simulink model "VCU_CS75_12_27_test"  (R2014a)
settings: Solver=FixedStepDiscrete  StartTime=0.0  StopTime=25  FixedStep=0.0005  RelTol=1e-3
undefined symbols (not defined in the file): D1, D2, D3, ecucoder_acal, ErrorSumMax1, ErrorSumMax2, ErrorSumMax3, I1, I2, I3, I_SW01_L, LaterlAngleCommand, LDW, P1, P2, P3, RemoteAcclPosition
libraries: simulink x913, ec5744lib x39
(part 22 of 30)

== system VCU_CS75_12_27_test/长安CS75底盘程序，20ms一次/Output/Subsystem/TransmitMessages3/ACC_3D5/ACC_RightTargetType ==
  ACC_RightTargetType : Inport
  ACC_RightTargetTypeRon : Rounding  Operator=round
  ACC_RightTargetType_1sat : Saturate  UpperLimit=224  LowerLimit=0
  ACC_RightTargetType_Convert : DataTypeConversion  OutDataTypeStr=uint8
  ACC_RightTargetType_Convert1 : DataTypeConversion  OutDataTypeStr=uint32
  ACC_RightTargetType_D : Product  Inputs=*/
  ACC_RightTargetType_F : Constant  OutDataTypeStr=single
  ACC_RightTargetType_L : simulink/Logic and Bit Operations/Bitwise Operator  logicop=AND  UseBitMask=on  BitMask=224  BitMaskRealWorld=Stored Integer
  ACC_RightTargetType_O : Constant  Value=0  OutDataTypeStr=single
  ACC_RightTargetType_S : ArithShift  BitShiftNumber=-5
  ACC_RightTargetType_sat : Saturate  UpperLimit=0  LowerLimit=0
  ACC_RightTargetType_st : Sum  Inputs=+-
  Constant{1..2,4..8} (7 alike) : Constant  Value=0  OutDataTypeStr=uint8
  output1 : Outport
  output2 : Outport  Port=2
  output3 : Outport  Port=3
  output4 : Outport  Port=4
  output5 : Outport  Port=5
  output6 : Outport  Port=6
  output7 : Outport  Port=7
  output8 : Outport  Port=8
  wires:
  ACC_RightTargetType/1 -> ACC_RightTargetType_sat/1
  ACC_RightTargetType_sat/1 -> ACC_RightTargetType_st/1
  ACC_RightTargetType_O/1 -> ACC_RightTargetType_st/2
  ACC_RightTargetType_st/1 -> ACC_RightTargetType_D/1
  ACC_RightTargetType_F/1 -> ACC_RightTargetType_D/2
  ACC_RightTargetType_D/1 -> ACC_RightTargetTypeRon/1
  ACC_RightTargetTypeRon/1 -> ACC_RightTargetType_S/1
  ACC_RightTargetType_S/1 -> ACC_RightTargetType_1sat/1
  ACC_RightTargetType_1sat/1 -> ACC_RightTargetType_Convert1/1
  ACC_RightTargetType_Convert1/1 -> ACC_RightTargetType_L/1
  ACC_RightTargetType_L/1 -> ACC_RightTargetType_Convert/1
  ACC_RightTargetType_Convert/1 -> output3/1
  Constant1/1 -> output1/1
  Constant2/1 -> output2/1
  Constant4/1 -> output4/1
  Constant5/1 -> output5/1
  Constant6/1 -> output6/1
  Constant7/1 -> output7/1
  Constant8/1 -> output8/1

== system VCU_CS75_12_27_test/长安CS75底盘程序，20ms一次/Output/Subsystem/TransmitMessages3/ACC_3D5/CRC ==
  CRC : Inport
  CRCRon : Rounding  Operator=round
  CRC_1sat : Saturate  UpperLimit=255  LowerLimit=0
  CRC_Convert : DataTypeConversion  OutDataTypeStr=uint8
  CRC_Convert1 : DataTypeConversion  OutDataTypeStr=uint32
  CRC_D : Product  Inputs=*/
  CRC_F : Constant  OutDataTypeStr=single
  CRC_L : simulink/Logic and Bit Operations/Bitwise Operator  logicop=AND  UseBitMask=on  BitMask=255  BitMaskRealWorld=Stored Integer
  CRC_O : Constant  Value=0  OutDataTypeStr=single
  CRC_S : ArithShift
  CRC_sat : Saturate  UpperLimit=0  LowerLimit=0
  CRC_st : Sum  Inputs=+-
  Constant{1..7} (7 alike) : Constant  Value=0  OutDataTypeStr=uint8
  output1 : Outport
  output2 : Outport  Port=2
  output3 : Outport  Port=3
  output4 : Outport  Port=4
  output5 : Outport  Port=5
  output6 : Outport  Port=6
  output7 : Outport  Port=7
  output8 : Outport  Port=8
  wires:
  CRC/1 -> CRC_sat/1
  CRC_sat/1 -> CRC_st/1
  CRC_O/1 -> CRC_st/2
  CRC_st/1 -> CRC_D/1
  CRC_F/1 -> CRC_D/2
  CRC_D/1 -> CRCRon/1
  CRCRon/1 -> CRC_S/1
  CRC_S/1 -> CRC_1sat/1
  CRC_1sat/1 -> CRC_Convert1/1
  CRC_Convert1/1 -> CRC_L/1
  CRC_L/1 -> CRC_Convert/1
  CRC_Convert/1 -> output8/1
  Constant1/1 -> output1/1
  Constant2/1 -> output2/1
  Constant3/1 -> output3/1
  Constant4/1 -> output4/1
  Constant5/1 -> output5/1
  Constant6/1 -> output6/1
  Constant7/1 -> output7/1

== system VCU_CS75_12_27_test/长安CS75底盘程序，20ms一次/Output/Subsystem/TransmitMessages3/ACC_3D5/RollingConter ==
  RollingConter : Inport
  Constant{1..6,8} (7 alike) : Constant  Value=0  OutDataTypeStr=uint8
  RollingConterRon : Rounding  Operator=round
  RollingConter_1sat : Saturate  UpperLimit=15  LowerLimit=0
  RollingConter_Convert : DataTypeConversion  OutDataTypeStr=uint8
  RollingConter_Convert1 : DataTypeConversion  OutDataTypeStr=uint32
  RollingConter_D : Product  Inputs=*/
  RollingConter_F : Constant  OutDataTypeStr=single
  RollingConter_L : simulink/Logic and Bit Operations/Bitwise Operator  logicop=AND  UseBitMask=on  BitMask=15  BitMaskRealWorld=Stored Integer
  RollingConter_O : Constant  Value=0  OutDataTypeStr=single
  RollingConter_S : ArithShift
  RollingConter_sat : Saturate  UpperLimit=0  LowerLimit=0
  RollingConter_st : Sum  Inputs=+-
  output1 : Outport
  output2 : Outport  Port=2
  output3 : Outport  Port=3
  output4 : Outport  Port=4
  output5 : Outport  Port=5
  output6 : Outport  Port=6
  output7 : Outport  Port=7
  output8 : Outport  Port=8
  wires:
  RollingConter/1 -> RollingConter_sat/1
  RollingConter_sat/1 -> RollingConter_st/1
  RollingConter_O/1 -> RollingConter_st/2
  RollingConter_st/1 -> RollingConter_D/1
  RollingConter_F/1 -> RollingConter_D/2
  RollingConter_D/1 -> RollingConterRon/1
  RollingConterRon/1 -> RollingConter_S/1
  RollingConter_S/1 -> RollingConter_1sat/1
  RollingConter_1sat/1 -> RollingConter_Convert1/1
  RollingConter_Convert1/1 -> RollingConter_L/1
  RollingConter_L/1 -> RollingConter_Convert/1
  RollingConter_Convert/1 -> output7/1
  Constant1/1 -> output1/1
  Constant2/1 -> output2/1
  Constant3/1 -> output3/1
  Constant4/1 -> output4/1
  Constant5/1 -> output5/1
  Constant6/1 -> output6/1
  Constant8/1 -> output8/1

== system VCU_CS75_12_27_test/长安CS75底盘程序，20ms一次/Output/Subsystem/TransmitMessages4/ACC_3E5/ACC_ACCObjEnableStatus ==
  ACC_ACCObjEnableStatus : Inport
  ACC_ACCObjEnableStatusRon : Rounding  Operator=round
  ACC_ACCObjEnableStatus_1sat : Saturate  UpperLimit=12  LowerLimit=0
  ACC_ACCObjEnableStatus_Convert : DataTypeConversion  OutDataTypeStr=uint8
  ACC_ACCObjEnableStatus_Convert1 : DataTypeConversion  OutDataTypeStr=uint32
  ACC_ACCObjEnableStatus_D : Product  Inputs=*/
  ACC_ACCObjEnableStatus_F : Constant  OutDataTypeStr=single
  ACC_ACCObjEnableStatus_L : simulink/Logic and Bit Operations/Bitwise Operator  logicop=AND  UseBitMask=on  BitMask=12  BitMaskRealWorld=Stored Integer
  ACC_ACCObjEnableStatus_O : Constant  Value=0  OutDataTypeStr=single
  ACC_ACCObjEnableStatus_S : ArithShift  BitShiftNumber=-2
  ACC_ACCObjEnableStatus_sat : Saturate  UpperLimit=0  LowerLimit=0
  ACC_ACCObjEnableStatus_st : Sum  Inputs=+-
  Constant{1..4,6..8} (7 alike) : Constant  Value=0  OutDataTypeStr=uint8
  output1 : Outport
  output2 : Outport  Port=2
  output3 : Outport  Port=3
  output4 : Outport  Port=4
  output5 : Outport  Port=5
  output6 : Outport  Port=6
  output7 : Outport  Port=7
  output8 : Outport  Port=8
  wires:
  Constant8/1 -> output8/1
  Constant7/1 -> output7/1
  Constant6/1 -> output6/1
  Constant4/1 -> output4/1
  Constant3/1 -> output3/1
  Constant2/1 -> output2/1
  Constant1/1 -> output1/1
  ACC_ACCObjEnableStatus_Convert/1 -> output5/1
  ACC_ACCObjEnableStatus_L/1 -> ACC_ACCObjEnableStatus_Convert/1
  ACC_ACCObjEnableStatus_Convert1/1 -> ACC_ACCObjEnableStatus_L/1
  ACC_ACCObjEnableStatus_1sat/1 -> ACC_ACCObjEnableStatus_Convert1/1
  ACC_ACCObjEnableStatus_S/1 -> ACC_ACCObjEnableStatus_1sat/1
  ACC_ACCObjEnableStatusRon/1 -> ACC_ACCObjEnableStatus_S/1
  ACC_ACCObjEnableStatus_D/1 -> ACC_ACCObjEnableStatusRon/1
  ACC_ACCObjEnableStatus_F/1 -> ACC_ACCObjEnableStatus_D/2
  ACC_ACCObjEnableStatus_st/1 -> ACC_ACCObjEnableStatus_D/1
  ACC_ACCObjEnableStatus_O/1 -> ACC_ACCObjEnableStatus_st/2
  ACC_ACCObjEnableStatus_sat/1 -> ACC_ACCObjEnableStatus_st/1
  ACC_ACCObjEnableStatus/1 -> ACC_ACCObjEnableStatus_sat/1

== system VCU_CS75_12_27_test/长安CS75底盘程序，20ms一次/Output/Subsystem/TransmitMessages4/ACC_3E5/ACC_AutoBrakeEnableStatus ==
  ACC_AutoBrakeEnableStatus : Inport
  ACC_AutoBrakeEnableStatusRon : Rounding  Operator=round
  ACC_AutoBrakeEnableStatus_1sat : Saturate  UpperLimit=128  LowerLimit=0
  ACC_AutoBrakeEnableStatus_Convert : DataTypeConversion  OutDataTypeStr=uint8
  ACC_AutoBrakeEnableStatus_Convert1 : DataTypeConversion  OutDataTypeStr=uint32
  ACC_AutoBrakeEnableStatus_D : Product  Inputs=*/
  ACC_AutoBrakeEnableStatus_F : Constant  OutDataTypeStr=single
  ACC_AutoBrakeEnableStatus_L : simulink/Logic and Bit Operations/Bitwise Operator  logicop=AND  UseBitMask=on  BitMask=128  BitMaskRealWorld=Stored Integer
  ACC_AutoBrakeEnableStatus_O : Constant  Value=0  OutDataTypeStr=single
  ACC_AutoBrakeEnableStatus_S : ArithShift  BitShiftNumber=-7
  ACC_AutoBrakeEnableStatus_sat : Saturate  UpperLimit=0  LowerLimit=0
  ACC_AutoBrakeEnableStatus_st : Sum  Inputs=+-
  Constant{1..6,8} (7 alike) : Constant  Value=0  OutDataTypeStr=uint8
  output1 : Outport
  output2 : Outport  Port=2
  output3 : Outport  Port=3
  output4 : Outport  Port=4
  output5 : Outport  Port=5
  output6 : Outport  Port=6
  output7 : Outport  Port=7
  output8 : Outport  Port=8
  wires:
  Constant8/1 -> output8/1
  Constant6/1 -> output6/1
  Constant5/1 -> output5/1
  Constant4/1 -> output4/1
  Constant3/1 -> output3/1
  Constant2/1 -> output2/1
  Constant1/1 -> output1/1
  ACC_AutoBrakeEnableStatus_Convert/1 -> output7/1
  ACC_AutoBrakeEnableStatus_L/1 -> ACC_AutoBrakeEnableStatus_Convert/1
  ACC_AutoBrakeEnableStatus_Convert1/1 -> ACC_AutoBrakeEnableStatus_L/1
  ACC_AutoBrakeEnableStatus_1sat/1 -> ACC_AutoBrakeEnableStatus_Convert1/1
  ACC_AutoBrakeEnableStatus_S/1 -> ACC_AutoBrakeEnableStatus_1sat/1
  ACC_AutoBrakeEnableStatusRon/1 -> ACC_AutoBrakeEnableStatus_S/1
  ACC_AutoBrakeEnableStatus_D/1 -> ACC_AutoBrakeEnableStatusRon/1
  ACC_AutoBrakeEnableStatus_F/1 -> ACC_AutoBrakeEnableStatus_D/2
  ACC_AutoBrakeEnableStatus_st/1 -> ACC_AutoBrakeEnableStatus_D/1
  ACC_AutoBrakeEnableStatus_O/1 -> ACC_AutoBrakeEnableStatus_st/2
  ACC_AutoBrakeEnableStatus_sat/1 -> ACC_AutoBrakeEnableStatus_st/1
  ACC_AutoBrakeEnableStatus/1 -> ACC_AutoBrakeEnableStatus_sat/1

== system VCU_CS75_12_27_test/长安CS75底盘程序，20ms一次/Output/Subsystem/TransmitMessages4/ACC_3E5/ACC_ControlType ==
  ACC_ControlType : Inport
  ACC_ControlTypeRon : Rounding  Operator=round
  ACC_ControlType_1sat : Saturate  UpperLimit=96  LowerLimit=0
  ACC_ControlType_Convert : DataTypeConversion  OutDataTypeStr=uint8
  ACC_ControlType_Convert1 : DataTypeConversion  OutDataTypeStr=uint32
  ACC_ControlType_D : Product  Inputs=*/
  ACC_ControlType_F : Constant  OutDataTypeStr=single
  ACC_ControlType_L : simulink/Logic and Bit Operations/Bitwise Operator  logicop=AND  UseBitMask=on  BitMask=96  BitMaskRealWorld=Stored Integer
  ACC_ControlType_O : Constant  Value=0  OutDataTypeStr=single
  ACC_ControlType_S : ArithShift  BitShiftNumber=-5
  ACC_ControlType_sat : Saturate  UpperLimit=0  LowerLimit=0
  ACC_ControlType_st : Sum  Inputs=+-
  Constant{1..2,4..8} (7 alike) : Constant  Value=0  OutDataTypeStr=uint8
  output1 : Outport
  output2 : Outport  Port=2
  output3 : Outport  Port=3
  output4 : Outport  Port=4
  output5 : Outport  Port=5
  output6 : Outport  Port=6
  output7 : Outport  Port=7
  output8 : Outport  Port=8
  wires:
  Constant8/1 -> output8/1
  Constant7/1 -> output7/1
  Constant6/1 -> output6/1
  Constant5/1 -> output5/1
  Constant4/1 -> output4/1
  Constant2/1 -> output2/1
  Constant1/1 -> output1/1
  ACC_ControlType_Convert/1 -> output3/1
  ACC_ControlType_L/1 -> ACC_ControlType_Convert/1
  ACC_ControlType_Convert1/1 -> ACC_ControlType_L/1
  ACC_ControlType_1sat/1 -> ACC_ControlType_Convert1/1
  ACC_ControlType_S/1 -> ACC_ControlType_1sat/1
  ACC_ControlTypeRon/1 -> ACC_ControlType_S/1
  ACC_ControlType_D/1 -> ACC_ControlTypeRon/1
  ACC_ControlType_F/1 -> ACC_ControlType_D/2
  ACC_ControlType_st/1 -> ACC_ControlType_D/1
  ACC_ControlType_O/1 -> ACC_ControlType_st/2
  ACC_ControlType_sat/1 -> ACC_ControlType_st/1
  ACC_ControlType/1 -> ACC_ControlType_sat/1

== system VCU_CS75_12_27_test/长安CS75底盘程序，20ms一次/Output/Subsystem/TransmitMessages4/ACC_3E5/ACC_DistanceTarObj ==
  ACC_DistanceTarObj : Inport
  ACC_DistanceTarObjRon : Rounding  Operator=round
  ACC_DistanceTarObj_1sat : Saturate  UpperLimit=224  LowerLimit=0
  ACC_DistanceTarObj_Convert : DataTypeConversion  OutDataTypeStr=uint8
  ACC_DistanceTarObj_Convert1 : DataTypeConversion  OutDataTypeStr=uint32
  ACC_DistanceTarObj_D : Product  Inputs=*/
  ACC_DistanceTarObj_F : Constant  OutDataTypeStr=single
  ACC_DistanceTarObj_L : simulink/Logic and Bit Operations/Bitwise Operator  logicop=AND  UseBitMask=on  BitMask=224  BitMaskRealWorld=Stored Integer
  ACC_DistanceTarObj_O : Constant  Value=0  OutDataTypeStr=single
  ACC_DistanceTarObj_S : ArithShift  BitShiftNumber=-5
  ACC_DistanceTarObj_sat : Saturate  UpperLimit=7  LowerLimit=0
  ACC_DistanceTarObj_st : Sum  Inputs=+-
  Constant{1,3..8} (7 alike) : Constant  Value=0  OutDataTypeStr=uint8
  output1 : Outport
  output2 : Outport  Port=2
  output3 : Outport  Port=3
  output4 : Outport  Port=4
  output5 : Outport  Port=5
  output6 : Outport  Port=6
  output7 : Outport  Port=7
  output8 : Outport  Port=8
  wires:
  Constant8/1 -> output8/1
  Constant7/1 -> output7/1
  Constant6/1 -> output6/1
  Constant5/1 -> output5/1
  Constant4/1 -> output4/1
  Constant3/1 -> output3/1
  Constant1/1 -> output1/1
  ACC_DistanceTarObj_Convert/1 -> output2/1
  ACC_DistanceTarObj_L/1 -> ACC_DistanceTarObj_Convert/1
  ACC_DistanceTarObj_Convert1/1 -> ACC_DistanceTarObj_L/1
  ACC_DistanceTarObj_1sat/1 -> ACC_DistanceTarObj_Convert1/1
  ACC_DistanceTarObj_S/1 -> ACC_DistanceTarObj_1sat/1
  ACC_DistanceTarObjRon/1 -> ACC_DistanceTarObj_S/1
  ACC_DistanceTarObj_D/1 -> ACC_DistanceTarObjRon/1
  ACC_DistanceTarObj_F/1 -> ACC_DistanceTarObj_D/2
  ACC_DistanceTarObj_st/1 -> ACC_DistanceTarObj_D/1
  ACC_DistanceTarObj_O/1 -> ACC_DistanceTarObj_st/2
  ACC_DistanceTarObj_sat/1 -> ACC_DistanceTarObj_st/1
  ACC_DistanceTarObj/1 -> ACC_DistanceTarObj_sat/1

== system VCU_CS75_12_27_test/长安CS75底盘程序，20ms一次/Output/Subsystem/TransmitMessages4/ACC_3E5/ACC_EPBReq ==
  ACC_EPBReq : Inport
  ACC_EPBReqRon : Rounding  Operator=round
  ACC_EPBReq_1sat : Saturate  UpperLimit=32  LowerLimit=0
  ACC_EPBReq_Convert : DataTypeConversion  OutDataTypeStr=uint8
  ACC_EPBReq_Convert1 : DataTypeConversion  OutDataTypeStr=uint32
  ACC_EPBReq_D : Product  Inputs=*/
  ACC_EPBReq_F : Constant  OutDataTypeStr=single
  ACC_EPBReq_L : simulink/Logic and Bit Operations/Bitwise Operator  logicop=AND  UseBitMask=on  BitMask=32  BitMaskRealWorld=Stored Integer
  ACC_EPBReq_O : Constant  Value=0  OutDataTypeStr=single
  ACC_EPBReq_S : ArithShift  BitShiftNumber=-5
  ACC_EPBReq_sat : Saturate  UpperLimit=0  LowerLimit=0
  ACC_EPBReq_st : Sum  Inputs=+-
  Constant{1..6,8} (7 alike) : Constant  Value=0  OutDataTypeStr=uint8
  output1 : Outport
  output2 : Outport  Port=2
  output3 : Outport  Port=3
  output4 : Outport  Port=4
  output5 : Outport  Port=5
  output6 : Outport  Port=6
  output7 : Outport  Port=7
  output8 : Outport  Port=8
  wires:
  Constant8/1 -> output8/1
  Constant6/1 -> output6/1
  Constant5/1 -> output5/1
  Constant4/1 -> output4/1
  Constant3/1 -> output3/1
  Constant2/1 -> output2/1
  Constant1/1 -> output1/1
  ACC_EPBReq_Convert/1 -> output7/1
  ACC_EPBReq_L/1 -> ACC_EPBReq_Convert/1
  ACC_EPBReq_Convert1/1 -> ACC_EPBReq_L/1
  ACC_EPBReq_1sat/1 -> ACC_EPBReq_Convert1/1
  ACC_EPBReq_S/1 -> ACC_EPBReq_1sat/1
  ACC_EPBReqRon/1 -> ACC_EPBReq_S/1
  ACC_EPBReq_D/1 -> ACC_EPBReqRon/1
  ACC_EPBReq_F/1 -> ACC_EPBReq_D/2
  ACC_EPBReq_st/1 -> ACC_EPBReq_D/1
  ACC_EPBReq_O/1 -> ACC_EPBReq_st/2
  ACC_EPBReq_sat/1 -> ACC_EPBReq_st/1
  ACC_EPBReq/1 -> ACC_EPBReq_sat/1

== system VCU_CS75_12_27_test/长安CS75底盘程序，20ms一次/Output/Subsystem/TransmitMessages4/ACC_3E5/ACC_FCWEnableStatus ==
  ACC_FCWEnableStatus : Inport
  ACC_FCWEnableStatusRon : Rounding  Operator=round
  ACC_FCWEnableStatus_1sat : Saturate  UpperLimit=1  LowerLimit=0
  ACC_FCWEnableStatus_Convert : DataTypeConversion  OutDataTypeStr=uint8
  ACC_FCWEnableStatus_Convert1 : DataTypeConversion  OutDataTypeStr=uint32
  ACC_FCWEnableStatus_D : Product  Inputs=*/
  ACC_FCWEnableStatus_F : Constant  OutDataTypeStr=single
  ACC_FCWEnableStatus_L : simulink/Logic and Bit Operations/Bitwise Operator  logicop=AND  UseBitMask=on  BitMask=1  BitMaskRealWorld=Stored Integer
  ACC_FCWEnableStatus_O : Constant  Value=0  OutDataTypeStr=single
  ACC_FCWEnableStatus_S : ArithShift
  ACC_FCWEnableStatus_sat : Saturate  UpperLimit=0  LowerLimit=0
  ACC_FCWEnableStatus_st : Sum  Inputs=+-
  Constant{1..5,7..8} (7 alike) : Constant  Value=0  OutDataTypeStr=uint8
  output1 : Outport
  output2 : Outport  Port=2
  output3 : Outport  Port=3
  output4 : Outport  Port=4
  output5 : Outport  Port=5
  output6 : Outport  Port=6
  output7 : Outport  Port=7
  output8 : Outport  Port=8
  wires:
  Constant8/1 -> output8/1
  Constant7/1 -> output7/1
  Constant5/1 -> output5/1
  Constant4/1 -> output4/1
  Constant3/1 -> output3/1
  Constant2/1 -> output2/1
  Constant1/1 -> output1/1
  ACC_FCWEnableStatus_Convert/1 -> output6/1
  ACC_FCWEnableStatus_L/1 -> ACC_FCWEnableStatus_Convert/1
  ACC_FCWEnableStatus_Convert1/1 -> ACC_FCWEnableStatus_L/1
  ACC_FCWEnableStatus_1sat/1 -> ACC_FCWEnableStatus_Convert1/1
  ACC_FCWEnableStatus_S/1 -> ACC_FCWEnableStatus_1sat/1
  ACC_FCWEnableStatusRon/1 -> ACC_FCWEnableStatus_S/1
  ACC_FCWEnableStatus_D/1 -> ACC_FCWEnableStatusRon/1
  ACC_FCWEnableStatus_F/1 -> ACC_FCWEnableStatus_D/2
  ACC_FCWEnableStatus_st/1 -> ACC_FCWEnableStatus_D/1
  ACC_FCWEnableStatus_O/1 -> ACC_FCWEnableStatus_st/2
  ACC_FCWEnableStatus_sat/1 -> ACC_FCWEnableStatus_st/1
  ACC_FCWEnableStatus/1 -> ACC_FCWEnableStatus_sat/1

== system VCU_CS75_12_27_test/长安CS75底盘程序，20ms一次/Output/Subsystem/TransmitMessages4/ACC_3E5/ACC_FCWSensityStatus ==
  ACC_FCWSensityStatus : Inport
  ACC_FCWSensityStatusRon : Rounding  Operator=round
  ACC_FCWSensityStatus_1sat : Saturate  UpperLimit=48  LowerLimit=0
  ACC_FCWSensityStatus_Convert : DataTypeConversion  OutDataTypeStr=uint8
  ACC_FCWSensityStatus_Convert1 : DataTypeConversion  OutDataTypeStr=uint32
  ACC_FCWSensityStatus_D : Product  Inputs=*/
  ACC_FCWSensityStatus_F : Constant  OutDataTypeStr=single
  ACC_FCWSensityStatus_L : simulink/Logic and Bit Operations/Bitwise Operator  logicop=AND  UseBitMask=on  BitMask=48  BitMaskRealWorld=Stored Integer
  ACC_FCWSensityStatus_O : Constant  Value=0  OutDataTypeStr=single
  ACC_FCWSensityStatus_S : ArithShift  BitShiftNumber=-4
  ACC_FCWSensityStatus_sat : Saturate  UpperLimit=3  LowerLimit=0
  ACC_FCWSensityStatus_st : Sum  Inputs=+-
  Constant{1..4,6..8} (7 alike) : Constant  Value=0  OutDataTypeStr=uint8
  output1 : Outport
  output2 : Outport  Port=2
  output3 : Outport  Port=3
  output4 : Outport  Port=4
  output5 : Outport  Port=5
  output6 : Outport  Port=6
  output7 : Outport  Port=7
  output8 : Outport  Port=8
  wires:
  Constant8/1 -> output8/1
  Constant7/1 -> output7/1
  Constant6/1 -> output6/1
  Constant4/1 -> output4/1
  Constant3/1 -> output3/1
  Constant2/1 -> output2/1
  Constant1/1 -> output1/1
  ACC_FCWSensityStatus_Convert/1 -> output5/1
  ACC_FCWSensityStatus_L/1 -> ACC_FCWSensityStatus_Convert/1
  ACC_FCWSensityStatus_Convert1/1 -> ACC_FCWSensityStatus_L/1
  ACC_FCWSensityStatus_1sat/1 -> ACC_FCWSensityStatus_Convert1/1
  ACC_FCWSensityStatus_S/1 -> ACC_FCWSensityStatus_1sat/1
  ACC_FCWSensityStatusRon/1 -> ACC_FCWSensityStatus_S/1
  ACC_FCWSensityStatus_D/1 -> ACC_FCWSensityStatusRon/1
  ACC_FCWSensityStatus_F/1 -> ACC_FCWSensityStatus_D/2
  ACC_FCWSensityStatus_st/1 -> ACC_FCWSensityStatus_D/1
  ACC_FCWSensityStatus_O/1 -> ACC_FCWSensityStatus_st/2
  ACC_FCWSensityStatus_sat/1 -> ACC_FCWSensityStatus_st/1
  ACC_FCWSensityStatus/1 -> ACC_FCWSensityStatus_sat/1

== system VCU_CS75_12_27_test/长安CS75底盘程序，20ms一次/Output/Subsystem/TransmitMessages4/ACC_3E5/ACC_ObjValid ==
  ACC_ObjValid : Inport
  ACC_ObjValidRon : Rounding  Operator=round
  ACC_ObjValid_1sat : Saturate  UpperLimit=2  LowerLimit=0
  ACC_ObjValid_Convert : DataTypeConversion  OutDataTypeStr=uint8
  ACC_ObjValid_Convert1 : DataTypeConversion  OutDataTypeStr=uint32
  ACC_ObjValid_D : Product  Inputs=*/
  ACC_ObjValid_F : Constant  OutDataTypeStr=single
  ACC_ObjValid_L : simulink/Logic and Bit Operations/Bitwise Operator  logicop=AND  UseBitMask=on  BitMask=2  BitMaskRealWorld=Stored Integer
  ACC_ObjValid_O : Constant  Value=0  OutDataTypeStr=single
  ACC_ObjValid_S : ArithShift  BitShiftNumber=-1
  ACC_ObjValid_sat : Saturate  UpperLimit=0  LowerLimit=0
  ACC_ObjValid_st : Sum  Inputs=+-
  Constant{1,3..8} (7 alike) : Constant  Value=0  OutDataTypeStr=uint8
  output1 : Outport
  output2 : Outport  Port=2
  output3 : Outport  Port=3
  output4 : Outport  Port=4
  output5 : Outport  Port=5
  output6 : Outport  Port=6
  output7 : Outport  Port=7
  output8 : Outport  Port=8
  wires:
  Constant8/1 -> output8/1
  Constant7/1 -> output7/1
  Constant6/1 -> output6/1
  Constant5/1 -> output5/1
  Constant4/1 -> output4/1
  Constant3/1 -> output3/1
  Constant1/1 -> output1/1
  ACC_ObjValid_Convert/1 -> output2/1
  ACC_ObjValid_L/1 -> ACC_ObjValid_Convert/1
  ACC_ObjValid_Convert1/1 -> ACC_ObjValid_L/1
  ACC_ObjValid_1sat/1 -> ACC_ObjValid_Convert1/1
  ACC_ObjValid_S/1 -> ACC_ObjValid_1sat/1
  ACC_ObjValidRon/1 -> ACC_ObjValid_S/1
  ACC_ObjValid_D/1 -> ACC_ObjValidRon/1
  ACC_ObjValid_F/1 -> ACC_ObjValid_D/2
  ACC_ObjValid_st/1 -> ACC_ObjValid_D/1
  ACC_ObjValid_O/1 -> ACC_ObjValid_st/2
  ACC_ObjValid_sat/1 -> ACC_ObjValid_st/1
  ACC_ObjValid/1 -> ACC_ObjValid_sat/1

== system VCU_CS75_12_27_test/长安CS75底盘程序，20ms一次/Output/Subsystem/TransmitMessages4/ACC_3E5/ACC_SetSpeedDisplay ==
  ACC_SetSpeedDisplay : Inport
  ACC_SetSpeedDisplayRon : Rounding  Operator=round
  ACC_SetSpeedDisplay_1sat : Saturate  UpperLimit=255  LowerLimit=0
  ACC_SetSpeedDisplay_Convert : DataTypeConversion  OutDataTypeStr=uint8
  ACC_SetSpeedDisplay_Convert1 : DataTypeConversion  OutDataTypeStr=uint32
  ACC_SetSpeedDisplay_D : Product  Inputs=*/
  ACC_SetSpeedDisplay_F : Constant  OutDataTypeStr=single
  ACC_SetSpeedDisplay_L : simulink/Logic and Bit Operations/Bitwise Operator  logicop=AND  UseBitMask=on  BitMask=255  BitMaskRealWorld=Stored Integer
  ACC_SetSpeedDisplay_O : Constant  Value=0  OutDataTypeStr=single
  ACC_SetSpeedDisplay_S : ArithShift
  ACC_SetSpeedDisplay_sat : Saturate  UpperLimit=255  LowerLimit=0
  ACC_SetSpeedDisplay_st : Sum  Inputs=+-
  Constant{2..8} (7 alike) : Constant  Value=0  OutDataTypeStr=uint8
  output1 : Outport
  output2 : Outport  Port=2
  output3 : Outport  Port=3
  output4 : Outport  Port=4
  output5 : Outport  Port=5
  output6 : Outport  Port=6
  output7 : Outport  Port=7
  output8 : Outport  Port=8
  wires:
  Constant8/1 -> output8/1
  Constant7/1 -> output7/1
  Constant6/1 -> output6/1
  Constant5/1 -> output5/1
  Constant4/1 -> output4/1
  Constant3/1 -> output3/1
  Constant2/1 -> output2/1
  ACC_SetSpeedDisplay_Convert/1 -> output1/1
  ACC_SetSpeedDisplay_L/1 -> ACC_SetSpeedDisplay_Convert/1
  ACC_SetSpeedDisplay_Convert1/1 -> ACC_SetSpeedDisplay_L/1
  ACC_SetSpeedDisplay_1sat/1 -> ACC_SetSpeedDisplay_Convert1/1
  ACC_SetSpeedDisplay_S/1 -> ACC_SetSpeedDisplay_1sat/1
  ACC_SetSpeedDisplayRon/1 -> ACC_SetSpeedDisplay_S/1
  ACC_SetSpeedDisplay_D/1 -> ACC_SetSpeedDisplayRon/1
  ACC_SetSpeedDisplay_F/1 -> ACC_SetSpeedDisplay_D/2
  ACC_SetSpeedDisplay_st/1 -> ACC_SetSpeedDisplay_D/1
  ACC_SetSpeedDisplay_O/1 -> ACC_SetSpeedDisplay_st/2
  ACC_SetSpeedDisplay_sat/1 -> ACC_SetSpeedDisplay_st/1
  ACC_SetSpeedDisplay/1 -> ACC_SetSpeedDisplay_sat/1

== system VCU_CS75_12_27_test/长安CS75底盘程序，20ms一次/Output/Subsystem/TransmitMessages4/ACC_3E5/ACC_TimeGapSet ==
  ACC_TimeGapSet : Inport
  ACC_TimeGapSetRon : Rounding  Operator=round
  ACC_TimeGapSet_1sat : Saturate  UpperLimit=28  LowerLimit=0
  ACC_TimeGapSet_Convert : DataTypeConversion  OutDataTypeStr=uint8
  ACC_TimeGapSet_Convert1 : DataTypeConversion  OutDataTypeStr=uint32
  ACC_TimeGapSet_D : Product  Inputs=*/
  ACC_TimeGapSet_F : Constant  OutDataTypeStr=single
  ACC_TimeGapSet_L : simulink/Logic and Bit Operations/Bitwise Operator  logicop=AND  UseBitMask=on  BitMask=28  BitMaskRealWorld=Stored Integer
  ACC_TimeGapSet_O : Constant  Value=0  OutDataTypeStr=single
  ACC_TimeGapSet_S : ArithShift  BitShiftNumber=-2
  ACC_TimeGapSet_sat : Saturate  UpperLimit=7  LowerLimit=0
  ACC_TimeGapSet_st : Sum  Inputs=+-
  Constant{1,3..8} (7 alike) : Constant  Value=0  OutDataTypeStr=uint8
  output1 : Outport
  output2 : Outport  Port=2
  output3 : Outport  Port=3
  output4 : Outport  Port=4
  output5 : Outport  Port=5
  output6 : Outport  Port=6
  output7 : Outport  Port=7
  output8 : Outport  Port=8
  wires:
  Constant8/1 -> output8/1
  Constant7/1 -> output7/1
  Constant6/1 -> output6/1
  Constant5/1 -> output5/1
  Constant4/1 -> output4/1
  Constant3/1 -> output3/1
  Constant1/1 -> output1/1
  ACC_TimeGapSet_Convert/1 -> output2/1
  ACC_TimeGapSet_L/1 -> ACC_TimeGapSet_Convert/1
  ACC_TimeGapSet_Convert1/1 -> ACC_TimeGapSet_L/1
  ACC_TimeGapSet_1sat/1 -> ACC_TimeGapSet_Convert1/1
  ACC_TimeGapSet_S/1 -> ACC_TimeGapSet_1sat/1
  ACC_TimeGapSetRon/1 -> ACC_TimeGapSet_S/1
  ACC_TimeGapSet_D/1 -> ACC_TimeGapSetRon/1
  ACC_TimeGapSet_F/1 -> ACC_TimeGapSet_D/2
  ACC_TimeGapSet_st/1 -> ACC_TimeGapSet_D/1
  ACC_TimeGapSet_O/1 -> ACC_TimeGapSet_st/2
  ACC_TimeGapSet_sat/1 -> ACC_TimeGapSet_st/1
  ACC_TimeGapSet/1 -> ACC_TimeGapSet_sat/1

== system VCU_CS75_12_27_test/长安CS75底盘程序，20ms一次/Output/Subsystem/TransmitMessages4/ACC_3E5/ACC_takeoverRequesr ==
  ACC_takeoverRequesr : Inport
  ACC_takeoverRequesrRon : Rounding  Operator=round
  ACC_takeoverRequesr_1sat : Saturate  UpperLimit=8  LowerLimit=0
  ACC_takeoverRequesr_Convert : DataTypeConversion  OutDataTypeStr=uint8
  ACC_takeoverRequesr_Convert1 : DataTypeConversion  OutDataTypeStr=uint32
  ACC_takeoverRequesr_D : Product  Inputs=*/
  ACC_takeoverRequesr_F : Constant  OutDataTypeStr=single
  ACC_takeoverRequesr_L : simulink/Logic and Bit Operations/Bitwise Operator  logicop=AND  UseBitMask=on  BitMask=8  BitMaskRealWorld=Stored Integer
  ACC_takeoverRequesr_O : Constant  Value=0  OutDataTypeStr=single
  ACC_takeoverRequesr_S : ArithShift  BitShiftNumber=-3
  ACC_takeoverRequesr_sat : Saturate  UpperLimit=1  LowerLimit=0
  ACC_takeoverRequesr_st : Sum  Inputs=+-
  Constant{1..3,5..8} (7 alike) : Constant  Value=0  OutDataTypeStr=uint8
  output1 : Outport
  output2 : Outport  Port=2
  output3 : Outport  Port=3
  output4 : Outport  Port=4
  output5 : Outport  Port=5
  output6 : Outport  Port=6
  output7 : Outport  Port=7
  output8 : Outport  Port=8
  wires:
  Constant8/1 -> output8/1
  Constant7/1 -> output7/1
  Constant6/1 -> output6/1
  Constant5/1 -> output5/1
  Constant3/1 -> output3/1
  Constant2/1 -> output2/1
  Constant1/1 -> output1/1
  ACC_takeoverRequesr_Convert/1 -> output4/1
  ACC_takeoverRequesr_L/1 -> ACC_takeoverRequesr_Convert/1
  ACC_takeoverRequesr_Convert1/1 -> ACC_takeoverRequesr_L/1
  ACC_takeoverRequesr_1sat/1 -> ACC_takeoverRequesr_Convert1/1
  ACC_takeoverRequesr_S/1 -> ACC_takeoverRequesr_1sat/1
  ACC_takeoverRequesrRon/1 -> ACC_takeoverRequesr_S/1
  ACC_takeoverRequesr_D/1 -> ACC_takeoverRequesrRon/1
  ACC_takeoverRequesr_F/1 -> ACC_takeoverRequesr_D/2
  ACC_takeoverRequesr_st/1 -> ACC_takeoverRequesr_D/1
  ACC_takeoverRequesr_O/1 -> ACC_takeoverRequesr_st/2
  ACC_takeoverRequesr_sat/1 -> ACC_takeoverRequesr_st/1
  ACC_takeoverRequesr/1 -> ACC_takeoverRequesr_sat/1

== system VCU_CS75_12_27_test/长安CS75底盘程序，20ms一次/Output/Subsystem/TransmitMessages4/ACC_3E5/CRC ==
  CRC : Inport
  CRCRon : Rounding  Operator=round
  CRC_1sat : Saturate  UpperLimit=255  LowerLimit=0
  CRC_Convert : DataTypeConversion  OutDataTypeStr=uint8
  CRC_Convert1 : DataTypeConversion  OutDataTypeStr=uint32
  CRC_D : Product  Inputs=*/
  CRC_F : Constant  OutDataTypeStr=single
  CRC_L : simulink/Logic and Bit Operations/Bitwise Operator  logicop=AND  UseBitMask=on  BitMask=255  BitMaskRealWorld=Stored Integer
  CRC_O : Constant  Value=0  OutDataTypeStr=single
  CRC_S : ArithShift
  CRC_sat : Saturate  UpperLimit=0  LowerLimit=0
  CRC_st : Sum  Inputs=+-
  Constant{1..7} (7 alike) : Constant  Value=0  OutDataTypeStr=uint8
  output1 : Outport
  output2 : Outport  Port=2
  output3 : Outport  Port=3
  output4 : Outport  Port=4
  output5 : Outport  Port=5
  output6 : Outport  Port=6
  output7 : Outport  Port=7
  output8 : Outport  Port=8
  wires:
  Constant7/1 -> output7/1
  Constant6/1 -> output6/1
  Constant5/1 -> output5/1
  Constant4/1 -> output4/1
  Constant3/1 -> output3/1
  Constant2/1 -> output2/1
  Constant1/1 -> output1/1
  CRC_Convert/1 -> output8/1
  CRC_L/1 -> CRC_Convert/1
  CRC_Convert1/1 -> CRC_L/1
  CRC_1sat/1 -> CRC_Convert1/1
  CRC_S/1 -> CRC_1sat/1
  CRCRon/1 -> CRC_S/1
  CRC_D/1 -> CRCRon/1
  CRC_F/1 -> CRC_D/2
  CRC_st/1 -> CRC_D/1
  CRC_O/1 -> CRC_st/2
  CRC_sat/1 -> CRC_st/1
  CRC/1 -> CRC_sat/1

== system VCU_CS75_12_27_test/长安CS75底盘程序，20ms一次/Output/Subsystem/TransmitMessages4/ACC_3E5/RollingConter ==
  RollingConter : Inport
  Constant{1..6,8} (7 alike) : Constant  Value=0  OutDataTypeStr=uint8
  RollingConterRon : Rounding  Operator=round
  RollingConter_1sat : Saturate  UpperLimit=15  LowerLimit=0
  RollingConter_Convert : DataTypeConversion  OutDataTypeStr=uint8
  RollingConter_Convert1 : DataTypeConversion  OutDataTypeStr=uint32
  RollingConter_D : Product  Inputs=*/
  RollingConter_F : Constant  OutDataTypeStr=single
  RollingConter_L : simulink/Logic and Bit Operations/Bitwise Operator  logicop=AND  UseBitMask=on  BitMask=15  BitMaskRealWorld=Stored Integer
  RollingConter_O : Constant  Value=0  OutDataTypeStr=single
  RollingConter_S : ArithShift
  RollingConter_sat : Saturate  UpperLimit=0  LowerLimit=0
  RollingConter_st : Sum  Inputs=+-
  output1 : Outport
  output2 : Outport  Port=2
  output3 : Outport  Port=3
  output4 : Outport  Port=4
  output5 : Outport  Port=5
  output6 : Outport  Port=6
  output7 : Outport  Port=7
  output8 : Outport  Port=8
  wires:
  Constant8/1 -> output8/1
  Constant6/1 -> output6/1
  Constant5/1 -> output5/1
  Constant4/1 -> output4/1
  Constant3/1 -> output3/1
  Constant2/1 -> output2/1
  Constant1/1 -> output1/1
  RollingConter_Convert/1 -> output7/1
  RollingConter_L/1 -> RollingConter_Convert/1
  RollingConter_Convert1/1 -> RollingConter_L/1
  RollingConter_1sat/1 -> RollingConter_Convert1/1
  RollingConter_S/1 -> RollingConter_1sat/1
  RollingConterRon/1 -> RollingConter_S/1
  RollingConter_D/1 -> RollingConterRon/1
  RollingConter_F/1 -> RollingConter_D/2
  RollingConter_st/1 -> RollingConter_D/1
  RollingConter_O/1 -> RollingConter_st/2
  RollingConter_sat/1 -> RollingConter_st/1
  RollingConter/1 -> RollingConter_sat/1

== system VCU_CS75_12_27_test/长安CS75底盘程序，20ms一次/Output/Subsystem/TransmitMessages5/ACC_3F5/ACC_AEBTargetLatRange ==
  ACC_AEBTargetLatRange : Inport
  ACC_AEBTargetLatRangeBitCov : DataTypeConversion  OutDataTypeStr=uint8
  ACC_AEBTargetLatRangeCOV : DataTypeConversion  OutDataTypeStr=uint8
  ACC_AEBTargetLatRangeRon : Rounding  Operator=round
  ACC_AEBTargetLatRange_1sat : Saturate  UpperLimit=16368  LowerLimit=0
  ACC_AEBTargetLatRange_And : simulink/Logic and Bit Operations/Bitwise Operator  logicop=AND  UseBitMask=off  NumInputPorts=2  BitMask=bin2dec('11011001')  BitMaskRealWorld=Stored Integer
  ACC_AEBTargetLatRange_And_C : Constant  Value=255  OutDataTypeStr=uint32
  ACC_AEBTargetLatRange_Convert : DataTypeConversion  OutDataTypeStr=uint32
  ACC_AEBTargetLatRange_D : Product  Inputs=*/
  ACC_AEBTargetLatRange_D1 : Product  Inputs=*/
  ACC_AEBTargetLatRange_F : Constant  Value=0.1  OutDataTypeStr=single
  ACC_AEBTargetLatRange_L : simulink/Logic and Bit Operations/Bitwise Operator  logicop=AND  UseBitMask=on  BitMask=16368  BitMaskRealWorld=Stored Integer
  ACC_AEBTargetLatRange_O : Constant  Value=-50  OutDataTypeStr=single
  ACC_AEBTargetLatRange_S : ArithShift  BitShiftNumber=-4
  ACC_AEBTargetLatRange_sat : Saturate  UpperLimit=52.3  LowerLimit=-50
  ACC_AEBTargetLatRange_st : Sum  Inputs=+-
  ACC_AEBTargetLatRangeoutput3_C : Constant  Value=256
  Constant{1..2,5..8} (6 alike) : Constant  Value=0  OutDataTypeStr=uint8
  output1 : Outport
  output2 : Outport  Port=2
  output3 : Outport  Port=3
  output4 : Outport  Port=4
  output5 : Outport  Port=5
  output6 : Outport  Port=6
  output7 : Outport  Port=7
  output8 : Outport  Port=8
  wires:
  ACC_AEBTargetLatRange/1 -> ACC_AEBTargetLatRange_sat/1
  ACC_AEBTargetLatRange_sat/1 -> ACC_AEBTargetLatRange_st/1
  ACC_AEBTargetLatRange_O/1 -> ACC_AEBTargetLatRange_st/2
  ACC_AEBTargetLatRange_st/1 -> ACC_AEBTargetLatRange_D/1
  ACC_AEBTargetLatRange_F/1 -> ACC_AEBTargetLatRange_D/2
  ACC_AEBTargetLatRange_D/1 -> ACC_AEBTargetLatRangeRon/1
  ACC_AEBTargetLatRangeRon/1 -> ACC_AEBTargetLatRange_S/1
  ACC_AEBTargetLatRange_S/1 -> ACC_AEBTargetLatRange_1sat/1
  ACC_AEBTargetLatRange_1sat/1 -> ACC_AEBTargetLatRange_Convert/1
  ACC_AEBTargetLatRange_Convert/1 -> ACC_AEBTargetLatRange_L/1
  ACC_AEBTargetLatRange_L/1 -> ACC_AEBTargetLatRange_D1/1, ACC_AEBTargetLatRange_And/1
  ACC_AEBTargetLatRangeoutput3_C/1 -> ACC_AEBTargetLatRange_D1/2
  ACC_AEBTargetLatRange_D1/1 -> ACC_AEBTargetLatRangeCOV/1
  ACC_AEBTargetLatRangeCOV/1 -> output3/1
  ACC_AEBTargetLatRange_And_C/1 -> ACC_AEBTargetLatRange_And/2
  ACC_AEBTargetLatRange_And/1 -> ACC_AEBTargetLatRangeBitCov/1
  ACC_AEBTargetLatRangeBitCov/1 -> output4/1
  Constant1/1 -> output1/1
  Constant2/1 -> output2/1
  Constant5/1 -> output5/1
  Constant6/1 -> output6/1
  Constant7/1 -> output7/1
  Constant8/1 -> output8/1

== system VCU_CS75_12_27_test/长安CS75底盘程序，20ms一次/Output/Subsystem/TransmitMessages5/ACC_3F5/ACC_AEBTargetLngRange ==
  ACC_AEBTargetLngRange : Inport
  ACC_AEBTargetLngRangeBitCov : DataTypeConversion  OutDataTypeStr=uint8
  ACC_AEBTargetLngRangeCOV : DataTypeConversion  OutDataTypeStr=uint8
  ACC_AEBTargetLngRangeRon : Rounding  Operator=round
  ACC_AEBTargetLngRange_1sat : Saturate  UpperLimit=65408  LowerLimit=0
  ACC_AEBTargetLngRange_And : simulink/Logic and Bit Operations/Bitwise Operator  logicop=AND  UseBitMask=off  NumInputPorts=2  BitMask=bin2dec('11011001')  BitMaskRealWorld=Stored Integer
  ACC_AEBTargetLngRange_And_C : Constant  Value=255  OutDataTypeStr=uint32
  ACC_AEBTargetLngRange_Convert : DataTypeConversion  OutDataTypeStr=uint32
  ACC_AEBTargetLngRange_D : Product  Inputs=*/
  ACC_AEBTargetLngRange_D1 : Product  Inputs=*/
  ACC_AEBTargetLngRange_F : Constant  Value=0.5  OutDataTypeStr=single
  ACC_AEBTargetLngRange_L : simulink/Logic and Bit Operations/Bitwise Operator  logicop=AND  UseBitMask=on  BitMask=65408  BitMaskRealWorld=Stored Integer
  ACC_AEBTargetLngRange_O : Constant  Value=0  OutDataTypeStr=single
  ACC_AEBTargetLngRange_S : ArithShift  BitShiftNumber=-7
  ACC_AEBTargetLngRange_sat : Saturate  UpperLimit=0  LowerLimit=0
  ACC_AEBTargetLngRange_st : Sum  Inputs=+-
  ACC_AEBTargetLngRangeoutput1_C : Constant  Value=256
  Constant{3..8} (6 alike) : Constant  Value=0  OutDataTypeStr=uint8
  output1 : Outport
  output2 : Outport  Port=2
  output3 : Outport  Port=3
  output4 : Outport  Port=4
  output5 : Outport  Port=5
  output6 : Outport  Port=6
  output7 : Outport  Port=7
  output8 : Outport  Port=8
  wires:
  ACC_AEBTargetLngRange/1 -> ACC_AEBTargetLngRange_sat/1
  ACC_AEBTargetLngRange_sat/1 -> ACC_AEBTargetLngRange_st/1
  ACC_AEBTargetLngRange_O/1 -> ACC_AEBTargetLngRange_st/2
  ACC_AEBTargetLngRange_st/1 -> ACC_AEBTargetLngRange_D/1
  ACC_AEBTargetLngRange_F/1 -> ACC_AEBTargetLngRange_D/2
  ACC_AEBTargetLngRange_D/1 -> ACC_AEBTargetLngRangeRon/1
  ACC_AEBTargetLngRangeRon/1 -> ACC_AEBTargetLngRange_S/1
  ACC_AEBTargetLngRange_S/1 -> ACC_AEBTargetLngRange_1sat/1
  ACC_AEBTargetLngRange_1sat/1 -> ACC_AEBTargetLngRange_Convert/1
  ACC_AEBTargetLngRange_Convert/1 -> ACC_AEBTargetLngRange_L/1
  ACC_AEBTargetLngRange_L/1 -> ACC_AEBTargetLngRange_D1/1, ACC_AEBTargetLngRange_And/1
  ACC_AEBTargetLngRangeoutput1_C/1 -> ACC_AEBTargetLngRange_D1/2
  ACC_AEBTargetLngRange_D1/1 -> ACC_AEBTargetLngRangeCOV/1
  ACC_AEBTargetLngRangeCOV/1 -> output1/1
  ACC_AEBTargetLngRange_And_C/1 -> ACC_AEBTargetLngRange_And/2
  ACC_AEBTargetLngRange_And/1 -> ACC_AEBTargetLngRangeBitCov/1
  ACC_AEBTargetLngRangeBitCov/1 -> output2/1
  Constant3/1 -> output3/1
  Constant4/1 -> output4/1
  Constant5/1 -> output5/1
  Constant6/1 -> output6/1
  Constant7/1 -> output7/1
  Constant8/1 -> output8/1

== system VCU_CS75_12_27_test/长安CS75底盘程序，20ms一次/Output/Subsystem/TransmitMessages5/ACC_3F5/ACC_AEBTargetRelSpeed ==
  ACC_AEBTargetRelSpeed : Inport
  ACC_AEBTargetRelSpeedBitCov : DataTypeConversion  OutDataTypeStr=uint8
  ACC_AEBTargetRelSpeedCOV : DataTypeConversion  OutDataTypeStr=uint8
  ACC_AEBTargetRelSpeedRon : Rounding  Operator=round
  ACC_AEBTargetRelSpeed_1sat : Saturate  UpperLimit=32704  LowerLimit=0
  ACC_AEBTargetRelSpeed_And : simulink/Logic and Bit Operations/Bitwise Operator  logicop=AND  UseBitMask=off  NumInputPorts=2  BitMask=bin2dec('11011001')  BitMaskRealWorld=Stored Integer
  ACC_AEBTargetRelSpeed_And_C : Constant  Value=255  OutDataTypeStr=uint32
  ACC_AEBTargetRelSpeed_Convert : DataTypeConversion  OutDataTypeStr=uint32
  ACC_AEBTargetRelSpeed_D : Product  Inputs=*/
  ACC_AEBTargetRelSpeed_D1 : Product  Inputs=*/
  ACC_AEBTargetRelSpeed_F : Constant  OutDataTypeStr=single
  ACC_AEBTargetRelSpeed_L : simulink/Logic and Bit Operations/Bitwise Operator  logicop=AND  UseBitMask=on  BitMask=32704  BitMaskRealWorld=Stored Integer
  ACC_AEBTargetRelSpeed_O : Constant  Value=0  OutDataTypeStr=single
  ACC_AEBTargetRelSpeed_S : ArithShift  BitShiftNumber=-6
  ACC_AEBTargetRelSpeed_sat : Saturate  UpperLimit=0  LowerLimit=0
  ACC_AEBTargetRelSpeed_st : Sum  Inputs=+-
  ACC_AEBTargetRelSpeedoutput2_C : Constant  Value=256
  Constant{1,4..8} (6 alike) : Constant  Value=0  OutDataTypeStr=uint8
  output1 : Outport
  output2 : Outport  Port=2
  output3 : Outport  Port=3
  output4 : Outport  Port=4
  output5 : Outport  Port=5
  output6 : Outport  Port=6
  output7 : Outport  Port=7
  output8 : Outport  Port=8
  wires:
  ACC_AEBTargetRelSpeed/1 -> ACC_AEBTargetRelSpeed_sat/1
  ACC_AEBTargetRelSpeed_sat/1 -> ACC_AEBTargetRelSpeed_st/1
  ACC_AEBTargetRelSpeed_O/1 -> ACC_AEBTargetRelSpeed_st/2
  ACC_AEBTargetRelSpeed_st/1 -> ACC_AEBTargetRelSpeed_D/1
  ACC_AEBTargetRelSpeed_F/1 -> ACC_AEBTargetRelSpeed_D/2
  ACC_AEBTargetRelSpeed_D/1 -> ACC_AEBTargetRelSpeedRon/1
  ACC_AEBTargetRelSpeedRon/1 -> ACC_AEBTargetRelSpeed_S/1
  ACC_AEBTargetRelSpeed_S/1 -> ACC_AEBTargetRelSpeed_1sat/1
  ACC_AEBTargetRelSpeed_1sat/1 -> ACC_AEBTargetRelSpeed_Convert/1
  ACC_AEBTargetRelSpeed_Convert/1 -> ACC_AEBTargetRelSpeed_L/1
  ACC_AEBTargetRelSpeed_L/1 -> ACC_AEBTargetRelSpeed_D1/1, ACC_AEBTargetRelSpeed_And/1
  ACC_AEBTargetRelSpeedoutput2_C/1 -> ACC_AEBTargetRelSpeed_D1/2
  ACC_AEBTargetRelSpeed_D1/1 -> ACC_AEBTargetRelSpeedCOV/1
  ACC_AEBTargetRelSpeedCOV/1 -> output2/1
  ACC_AEBTargetRelSpeed_And_C/1 -> ACC_AEBTargetRelSpeed_And/2
  ACC_AEBTargetRelSpeed_And/1 -> ACC_AEBTargetRelSpeedBitCov/1
  ACC_AEBTargetRelSpeedBitCov/1 -> output3/1
  Constant1/1 -> output1/1
  Constant4/1 -> output4/1
  Constant5/1 -> output5/1
  Constant6/1 -> output6/1
  Constant7/1 -> output7/1
  Constant8/1 -> output8/1

== system VCU_CS75_12_27_test/长安CS75底盘程序，20ms一次/Output/Subsystem/TransmitMessages5/ACC_3F5/ACC_HostPotentialTargetDetection ==
  ACC_HostPotentialTargetDetection : Inport
  ACC_HostPotentialTargetDetectionRon : Rounding  Operator=round
  ACC_HostPotentialTargetDetection_1sat : Saturate  UpperLimit=12  LowerLimit=0
  ACC_HostPotentialTargetDetection_Convert : DataTypeConversion  OutDataTypeStr=uint8
  ACC_HostPotentialTargetDetection_Convert1 : DataTypeConversion  OutDataTypeStr=uint32
  ACC_HostPotentialTargetDetection_D : Product  Inputs=*/
  ACC_HostPotentialTargetDetection_F : Constant  OutDataTypeStr=single
  ACC_HostPotentialTargetDetection_L : simulink/Logic and Bit Operations/Bitwise Operator  logicop=AND  UseBitMask=on  BitMask=12  BitMaskRealWorld=Stored Integer
  ACC_HostPotentialTargetDetection_O : Constant  Value=0  OutDataTypeStr=single
  ACC_HostPotentialTargetDetection_S : ArithShift  BitShiftNumber=-2
  ACC_HostPotentialTargetDetection_sat : Saturate  UpperLimit=3  LowerLimit=0
  ACC_HostPotentialTargetDetection_st : Sum  Inputs=+-
  Constant{1..3,5..8} (7 alike) : Constant  Value=0  OutDataTypeStr=uint8
  output1 : Outport
  output2 : Outport  Port=2
  output3 : Outport  Port=3
  output4 : Outport  Port=4
  output5 : Outport  Port=5
  output6 : Outport  Port=6
  output7 : Outport  Port=7
  output8 : Outport  Port=8
  wires:
  ACC_HostPotentialTargetDetection/1 -> ACC_HostPotentialTargetDetection_sat/1
  ACC_HostPotentialTargetDetection_sat/1 -> ACC_HostPotentialTargetDetection_st/1
  ACC_HostPotentialTargetDetection_O/1 -> ACC_HostPotentialTargetDetection_st/2
  ACC_HostPotentialTargetDetection_st/1 -> ACC_HostPotentialTargetDetection_D/1
  ACC_HostPotentialTargetDetection_F/1 -> ACC_HostPotentialTargetDetection_D/2
  ACC_HostPotentialTargetDetection_D/1 -> ACC_HostPotentialTargetDetectionRon/1
  ACC_HostPotentialTargetDetectionRon/1 -> ACC_HostPotentialTargetDetection_S/1
  ACC_HostPotentialTargetDetection_S/1 -> ACC_HostPotentialTargetDetection_1sat/1
  ACC_HostPotentialTargetDetection_1sat/1 -> ACC_HostPotentialTargetDetection_Convert1/1
  ACC_HostPotentialTargetDetection_Convert1/1 -> ACC_HostPotentialTargetDetection_L/1
  ACC_HostPotentialTargetDetection_L/1 -> ACC_HostPotentialTargetDetection_Convert/1
  ACC_HostPotentialTargetDetection_Convert/1 -> output4/1
  Constant1/1 -> output1/1
  Constant2/1 -> output2/1
  Constant3/1 -> output3/1
  Constant5/1 -> output5/1
  Constant6/1 -> output6/1
  Constant7/1 -> output7/1
  Constant8/1 -> output8/1

== system VCU_CS75_12_27_test/长安CS75底盘程序，20ms一次/Output/Subsystem/TransmitMessages5/ACC_3F5/ACC_HostPotentialTargetLatRng ==
  ACC_HostPotentialTargetLatRng : Inport
  ACC_HostPotentialTargetLatRngBitCov : DataTypeConversion  OutDataTypeStr=uint8
  ACC_HostPotentialTargetLatRngCOV : DataTypeConversion  OutDataTypeStr=uint8
  ACC_HostPotentialTargetLatRngRon : Rounding  Operator=round
  ACC_HostPotentialTargetLatRng_1sat : Saturate  UpperLimit=1023  LowerLimit=0
  ACC_HostPotentialTargetLatRng_And : simulink/Logic and Bit Operations/Bitwise Operator  logicop=AND  UseBitMask=off  NumInputPorts=2  BitMask=bin2dec('11011001')  BitMaskRealWorld=Stored Integer
  ACC_HostPotentialTargetLatRng_And_C : Constant  Value=255  OutDataTypeStr=uint32
  ACC_HostPotentialTargetLatRng_Convert : DataTypeConversion  OutDataTypeStr=uint32
  ACC_HostPotentialTargetLatRng_D : Product  Inputs=*/
  ACC_HostPotentialTargetLatRng_D1 : Product  Inputs=*/
  ACC_HostPotentialTargetLatRng_F : Constant  Value=0.1  OutDataTypeStr=single
  ACC_HostPotentialTargetLatRng_L : simulink/Logic and Bit Operations/Bitwise Operator  logicop=AND  UseBitMask=on  BitMask=1023  BitMaskRealWorld=Stored Integer
  ACC_HostPotentialTargetLatRng_O : Constant  Value=-50  OutDataTypeStr=single
  ACC_HostPotentialTargetLatRng_S : ArithShift
  ACC_HostPotentialTargetLatRng_sat : Saturate  UpperLimit=52.3  LowerLimit=-50
  ACC_HostPotentialTargetLatRng_st : Sum  Inputs=+-
  ACC_HostPotentialTargetLatRngoutput4_C : Constant  Value=256
  Constant{1..3,6..8} (6 alike) : Constant  Value=0  OutDataTypeStr=uint8
  output1 : Outport
  output2 : Outport  Port=2
  output3 : Outport  Port=3
  output4 : Outport  Port=4
  output5 : Outport  Port=5
  output6 : Outport  Port=6
  output7 : Outport  Port=7
  output8 : Outport  Port=8
  wires:
  ACC_HostPotentialTargetLatRng/1 -> ACC_HostPotentialTargetLatRng_sat/1
  ACC_HostPotentialTargetLatRng_sat/1 -> ACC_HostPotentialTargetLatRng_st/1
  ACC_HostPotentialTargetLatRng_O/1 -> ACC_HostPotentialTargetLatRng_st/2
  ACC_HostPotentialTargetLatRng_st/1 -> ACC_HostPotentialTargetLatRng_D/1
  ACC_HostPotentialTargetLatRng_F/1 -> ACC_HostPotentialTargetLatRng_D/2
  ACC_HostPotentialTargetLatRng_D/1 -> ACC_HostPotentialTargetLatRngRon/1
  ACC_HostPotentialTargetLatRngRon/1 -> ACC_HostPotentialTargetLatRng_S/1
  ACC_HostPotentialTargetLatRng_S/1 -> ACC_HostPotentialTargetLatRng_1sat/1
  ACC_HostPotentialTargetLatRng_1sat/1 -> ACC_HostPotentialTargetLatRng_Convert/1
  ACC_HostPotentialTargetLatRng_Convert/1 -> ACC_HostPotentialTargetLatRng_L/1
  ACC_HostPotentialTargetLatRng_L/1 -> ACC_HostPotentialTargetLatRng_D1/1, ACC_HostPotentialTargetLatRng_And/1
  ACC_HostPotentialTargetLatRngoutput4_C/1 -> ACC_HostPotentialTargetLatRng_D1/2
  ACC_HostPotentialTargetLatRng_D1/1 -> ACC_HostPotentialTargetLatRngCOV/1
  ACC_HostPotentialTargetLatRngCOV/1 -> output4/1
  ACC_HostPotentialTargetLatRng_And_C/1 -> ACC_HostPotentialTargetLatRng_And/2
  ACC_HostPotentialTargetLatRng_And/1 -> ACC_HostPotentialTargetLatRngBitCov/1
  ACC_HostPotentialTargetLatRngBitCov/1 -> output5/1
  Constant1/1 -> output1/1
  Constant2/1 -> output2/1
  Constant3/1 -> output3/1
  Constant6/1 -> output6/1
  Constant7/1 -> output7/1
  Constant8/1 -> output8/1

== system VCU_CS75_12_27_test/长安CS75底盘程序，20ms一次/Output/Subsystem/TransmitMessages5/ACC_3F5/ACC_HostPotentialTargetLngRng ==
  ACC_HostPotentialTargetLngRng : Inport
  ACC_HostPotentialTargetLngRngBitCov : DataTypeConversion  OutDataTypeStr=uint8
  ACC_HostPotentialTargetLngRngCOV : DataTypeConversion  OutDataTypeStr=uint8
  ACC_HostPotentialTargetLngRngRon : Rounding  Operator=round
  ACC_HostPotentialTargetLngRng_1sat : Saturate  UpperLimit=65408  LowerLimit=0
  ACC_HostPotentialTargetLngRng_And : simulink/Logic and Bit Operations/Bitwise Operator  logicop=AND  UseBitMask=off  NumInputPorts=2  BitMask=bin2dec('11011001')  BitMaskRealWorld=Stored Integer
  ACC_HostPotentialTargetLngRng_And_C : Constant  Value=255  OutDataTypeStr=uint32
  ACC_HostPotentialTargetLngRng_Convert : DataTypeConversion  OutDataTypeStr=uint32
  ACC_HostPotentialTargetLngRng_D : Product  Inputs=*/
  ACC_HostPotentialTargetLngRng_D1 : Product  Inputs=*/
  ACC_HostPotentialTargetLngRng_F : Constant  Value=0.5  OutDataTypeStr=single
  ACC_HostPotentialTargetLngRng_L : simulink/Logic and Bit Operations/Bitwise Operator  logicop=AND  UseBitMask=on  BitMask=65408  BitMaskRealWorld=Stored Integer
  ACC_HostPotentialTargetLngRng_O : Constant  Value=0  OutDataTypeStr=single
  ACC_HostPotentialTargetLngRng_S : ArithShift  BitShiftNumber=-7
  ACC_HostPotentialTargetLngRng_sat : Saturate  UpperLimit=255.5  LowerLimit=0
  ACC_HostPotentialTargetLngRng_st : Sum  Inputs=+-
  ACC_HostPotentialTargetLngRngoutput6_C : Constant  Value=256
  Constant{1..5,8} (6 alike) : Constant  Value=0  OutDataTypeStr=uint8
  output1 : Outport
  output2 : Outport  Port=2
  output3 : Outport  Port=3
  output4 : Outport  Port=4
  output5 : Outport  Port=5
  output6 : Outport  Port=6
  output7 : Outport  Port=7
  output8 : Outport  Port=8
  wires:
  ACC_HostPotentialTargetLngRng/1 -> ACC_HostPotentialTargetLngRng_sat/1
  ACC_HostPotentialTargetLngRng_sat/1 -> ACC_HostPotentialTargetLngRng_st/1
  ACC_HostPotentialTargetLngRng_O/1 -> ACC_HostPotentialTargetLngRng_st/2
  ACC_HostPotentialTargetLngRng_st/1 -> ACC_HostPotentialTargetLngRng_D/1
  ACC_HostPotentialTargetLngRng_F/1 -> ACC_HostPotentialTargetLngRng_D/2
  ACC_HostPotentialTargetLngRng_D/1 -> ACC_HostPotentialTargetLngRngRon/1
  ACC_HostPotentialTargetLngRngRon/1 -> ACC_HostPotentialTargetLngRng_S/1
  ACC_HostPotentialTargetLngRng_S/1 -> ACC_HostPotentialTargetLngRng_1sat/1
  ACC_HostPotentialTargetLngRng_1sat/1 -> ACC_HostPotentialTargetLngRng_Convert/1
  ACC_HostPotentialTargetLngRng_Convert/1 -> ACC_HostPotentialTargetLngRng_L/1
  ACC_HostPotentialTargetLngRng_L/1 -> ACC_HostPotentialTargetLngRng_D1/1, ACC_HostPotentialTargetLngRng_And/1
  ACC_HostPotentialTargetLngRngoutput6_C/1 -> ACC_HostPotentialTargetLngRng_D1/2
  ACC_HostPotentialTargetLngRng_D1/1 -> ACC_HostPotentialTargetLngRngCOV/1
  ACC_HostPotentialTargetLngRngCOV/1 -> output6/1
  ACC_HostPotentialTargetLngRng_And_C/1 -> ACC_HostPotentialTargetLngRng_And/2
  ACC_HostPotentialTargetLngRng_And/1 -> ACC_HostPotentialTargetLngRngBitCov/1
  ACC_HostPotentialTargetLngRngBitCov/1 -> output7/1
  Constant1/1 -> output1/1
  Constant2/1 -> output2/1
  Constant3/1 -> output3/1
  Constant4/1 -> output4/1
  Constant5/1 -> output5/1
  Constant8/1 -> output8/1
